simulink model "cascaded_h_bridge_5_level"  (R2015b)
settings: Solver=VariableStepAuto  StartTime=0.0  StopTime=10.0  RelTol=1e-3
libraries: powerlib x18, simulink x8, powerlib_meascontrol x1
settings Model: Creator=hakan  LastModifiedBy=hakan

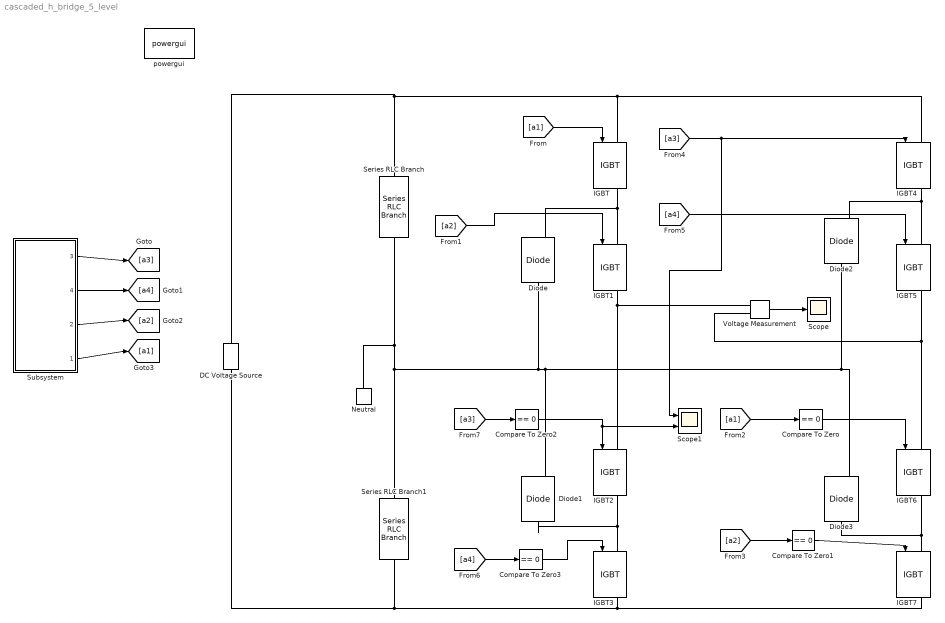
== system cascaded_h_bridge_5_level ==
  Compare To Zero{,1..3} (4 alike) : simulink/Logic and Bit Operations/Compare To Zero  relop===  OutDataTypeStr=boolean
  DC Voltage Source : powerlib/Electrical Sources/DC Voltage Source  Amplitude=100  Measurements=None
  Diode{,1..3} (4 alike) : powerlib/Power Electronics/Diode  Ron=0.001  Lon=0  Vf=0.8  IC=0  UseSnubber=off  Rs=500  Cs=250e-9  Measurements=on
  IGBT{,1..7} (8 alike) : powerlib/Power Electronics/IGBT  Ron=0.001  Lon=0  Vf=1  Tf=1e-6  Tt=2e-6  IC=0  Rs=1e5  Cs=inf  Measurements=on
  Neutral : powerlib/Elements/Neutral  LConnTagsString=a  NodeNumber=10
  Scope : Scope
  Scope1 : Scope  NumInputPorts=2
  Series RLC Branch : powerlib/Elements/Series RLC Branch  LConnTagsString=__new0  RConnTagsString=__new0  BranchType=RC  Resistance=1  Inductance=1e-3  SetiL0=off  InitialCurrent=0  Capacitance=1000e-6  Setx0=off  InitialVoltage=0  Measurements=None
  Series RLC Branch1 : powerlib/Elements/Series RLC Branch  LConnTagsString=__new0  RConnTagsString=__new0  BranchType=RC  Resistance=1  Inductance=1e-3  SetiL0=off  InitialCurrent=0  Capacitance=1000e-6  Setx0=off  InitialVoltage=0  Measurements=None
  Subsystem : Subsystem
  Voltage Measurement : powerlib/Measurements/Voltage Measurement  PhasorSimulation=off  OutputType=Complex  PSBequivalent=0
  powergui : powerlib/powergui  Priority=1  SimulationMode=Continuous  SolverType=Tustin/Backward Euler (TBE)  SampleTime=50e-6  frequency=60  SPID=off  DisableSnubberDevices=off  DisableRonSwitches=off  DisableVfSwitches=off  SwTol=0  DisplayEquations=off  Interpol=off  ExternalGateDelay=off  methode=off  Ts=10  FunctionMessages=off  echomessages=off  HookPort=off  EnableUseOfTLC=off  x0status=blocks  frequencyindice=0  Pbase=100e6  ErrMax=1e-4  Iterations=50  UnitsV=kV  UnitsW=MW  buscounter=0  RestoreLinks=warning  ResistiveCurrentMeasurement=off  Frange=[0:2:500]  Ylog=off  Xlog=on  ShowGrid=off  save=off  variable=ZData  structure=0  ZoomFFT=off  StartTime=0.0  cycles=1  DisplayStyle=1  fundamental=60  FreqAxis=off  MaxFrequency=1000  frequencyindicesteady=1  RmsSteady=1  display=off
  wires:
  Voltage Measurement/1 -> Scope/1
  Subsystem/1(3) -> [a3]
  Subsystem/2(4) -> [a4]
  Subsystem/3(2) -> [a2]
  Subsystem/4(1) -> [a1]
  [a1] -> IGBT/1
  [a2] -> IGBT1/1
  [a1] -> Compare To Zero/1
  Compare To Zero/1 -> IGBT6/1
  [a2] -> Compare To Zero1/1
  Compare To Zero1/1 -> IGBT7/1
  [a3] -> Scope1/1, IGBT4/1
  [a4] -> IGBT5/1
  [a3] -> Compare To Zero2/1
  Compare To Zero2/1 -> Scope1/2, IGBT2/1
  [a4] -> Compare To Zero3/1
  Compare To Zero3/1 -> IGBT3/1
  connections:
  IGBT/RConn1 -- Diode/RConn1 -- IGBT1/LConn1
  IGBT2/RConn1 -- Diode1/LConn1 -- IGBT3/LConn1
  IGBT4/RConn1 -- Diode2/RConn1 -- IGBT5/LConn1
  IGBT6/RConn1 -- Diode3/LConn1 -- IGBT7/LConn1
  Diode3/RConn1 -- Neutral/LConn1 -- Series RLC Branch/RConn1 -- Series RLC Branch1/LConn1 -- Diode/LConn1 -- Diode1/RConn1 -- Diode2/LConn1
  DC Voltage Source/RConn1 -- IGBT4/LConn1 -- IGBT/LConn1 -- Series RLC Branch/LConn1
  DC Voltage Source/LConn1 -- IGBT7/RConn1 -- IGBT3/RConn1 -- Series RLC Branch1/RConn1
  IGBT1/RConn1 -- IGBT2/LConn1 -- Voltage Measurement/LConn1
  IGBT5/RConn1 -- Voltage Measurement/LConn2 -- IGBT6/LConn1

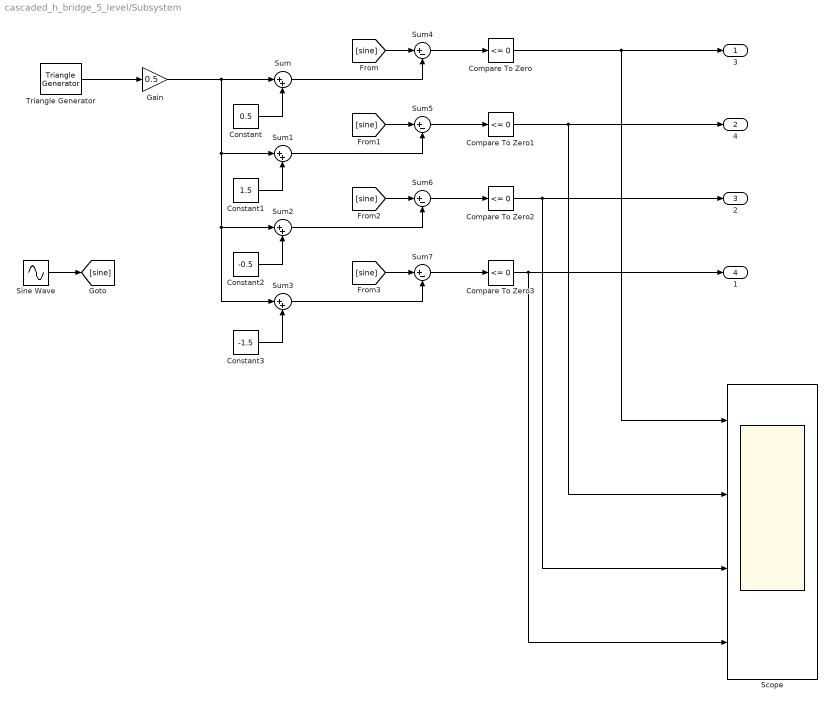
== system cascaded_h_bridge_5_level/Subsystem ==
  Compare To Zero{,1..3} (4 alike) : simulink/Logic and Bit Operations/Compare To Zero  relop=<=  OutDataTypeStr=boolean
  Constant : Constant  Value=0.5
  Constant1 : Constant  Value=1.5
  Constant2 : Constant  Value=-0.5
  Constant3 : Constant  Value=-1.5
  Gain : Gain  Gain=0.5
  Scope : Scope  NumInputPorts=4
  Sine Wave : Sin  Amplitude=2.5  Frequency=100*pi  SampleTime=0
  Sum{,1..3} (4 alike) : Sum  Inputs=|++
  Sum{4..7} (4 alike) : Sum  Inputs=|+-
  Triangle Generator : powerlib_meascontrol/Pulse & Signal Generators/Triangle Generator  Freq=2000  Phase=0  Ts=0
  3 : Outport
  4 : Outport  Port=2
  2 : Outport  Port=3
  1 : Outport  Port=4
  wires:
  Sum7/1 -> Compare To Zero3/1
  Constant1/1 -> Sum1/2
  Constant2/1 -> Sum2/2
  Triangle Generator/1 -> Gain/1
  Gain/1 -> Sum3/1, Sum2/1, Sum1/1, Sum/1
  Sine Wave/1 -> [sine]
  Constant/1 -> Sum/2
  Constant3/1 -> Sum3/2
  Sum1/1 -> Sum5/2
  Sum2/1 -> Sum6/2
  [sine] -> Sum5/1
  Compare To Zero3/1 -> 1/1, Scope/4
  Sum3/1 -> Sum7/2
  Sum4/1 -> Compare To Zero/1
  Sum5/1 -> Compare To Zero1/1
  Sum6/1 -> Compare To Zero2/1
  [sine] -> Sum4/1
  [sine] -> Sum7/1
  Sum/1 -> Sum4/2
  Compare To Zero1/1 -> 4/1, Scope/2
  Compare To Zero2/1 -> 2/1, Scope/3
  Compare To Zero/1 -> 3/1, Scope/1
  [sine] -> Sum6/1
